simulink model "FusionMODEL_version4"  (R2018a)
settings: Solver=FixedStepAuto  StartTime=0.0  StopTime=SimulationTime  FixedStep=SamplingTime  RelTol=1e-3
values from neighbouring files (symbols this model uses):
  ValidateGRID = true    [SensorFusion_Script0_main.m]
  ValidateLAYOUT = true    [SensorFusion_Script0_main.m]
  VisualizeCLUSTERING = true    [SensorFusion_Script0_main.m]
undefined symbols (not defined in the file or in its folder): ACTIVATE_CAM, ACTIVATE_RAD, CAM1_detTimeStamp, CAM1_MeasNoise, CAM1_objClassID, CAM1_PX, CAM1_PY, CAM1_VX, CAM1_VY, CAM2_detTimeStamp, CAM2_MeasNoise, CAM2_objClassID, CAM2_PX, CAM2_PY, CAM2_VX, CAM2_VY, CAM3_detTimeStamp, CAM3_MeasNoise, CAM3_objClassID, CAM3_PX, CAM3_PY, CAM3_VX, CAM3_VY, CAM4_detTimeStamp, CAM4_MeasNoise, CAM4_objClassID, CAM4_PX, CAM4_PY, CAM4_VX, CAM4_VY, CAM5_detTimeStamp, CAM5_MeasNoise, CAM5_objClassID, CAM5_PX, CAM5_PY, CAM5_VX, CAM5_VY, CAM6_detTimeStamp, CAM6_MeasNoise, CAM6_objClassID, CAM6_PX, CAM6_PY, CAM6_VX, CAM6_VY, CAM7_detTimeStamp, CAM7_MeasNoise, CAM7_objClassID, CAM7_PX, CAM7_PY, CAM7_VX, CAM7_VY, CAM8_detTimeStamp, CAM8_MeasNoise, CAM8_objClassID, CAM8_PX, CAM8_PY, CAM8_VX, CAM8_VY, CAM_nMeas, CAM_TYPE ... (+171)
libraries: simulink_extras x4
(part 1 of 9)
settings Model: SimulationMode=accelerator  Creator=Udit Bhaskar  LastModifiedBy=Udit Bhaskar
settings OptimizationCC: EfficientMapNaN2IntZero=off
settings HardwareCC: TargetBitPerPointer=64  TargetBitPerSizeT=64  TargetBitPerPtrDiffT=64  TargetLongLongMode=on  TargetIntDivRoundTo=Zero  TargetEndianess=LittleEndian  TargetWordSize=64  TargetHWDeviceType=MATLAB Host  ProdEqTarget=off
settings CodeAppCC: MaxIdLength=128
settings GRTTargetCC: TargetLangStandard=C89/C90 (ANSI)  CombineOutputUpdateFcns=off  GRTInterface=on

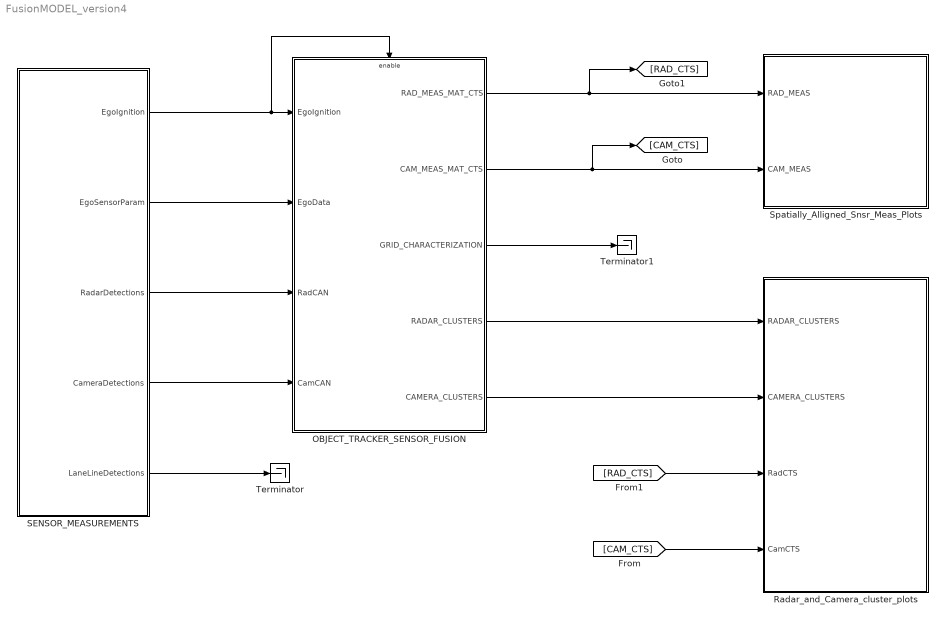
== system FusionMODEL_version4 ==
  OBJECT_TRACKER_SENSOR_FUSION : Subsystem
  Radar_and_Camera_cluster_plots : Subsystem
  SENSOR_MEASUREMENTS : Subsystem
  Spatially_Alligned_Snsr_Meas_Plots : Subsystem
  Terminator : Terminator
  Terminator1 : Terminator
  wires:
  SENSOR_MEASUREMENTS/5(LaneLineDetections) -> Terminator/1
  SENSOR_MEASUREMENTS/3(RadarDetections) -> OBJECT_TRACKER_SENSOR_FUSION/3(RadCAN)
  SENSOR_MEASUREMENTS/4(CameraDetections) -> OBJECT_TRACKER_SENSOR_FUSION/4(CamCAN)
  OBJECT_TRACKER_SENSOR_FUSION/1(RAD_MEAS_MAT_CTS) -> [RAD_CTS], Spatially_Alligned_Snsr_Meas_Plots/1(RAD_MEAS)
  OBJECT_TRACKER_SENSOR_FUSION/2(CAM_MEAS_MAT_CTS) -> [CAM_CTS], Spatially_Alligned_Snsr_Meas_Plots/2(CAM_MEAS)
  OBJECT_TRACKER_SENSOR_FUSION/3(GRID_CHARACTERIZATION) -> Terminator1/1
  SENSOR_MEASUREMENTS/1(EgoIgnition) -> OBJECT_TRACKER_SENSOR_FUSION/Enable, OBJECT_TRACKER_SENSOR_FUSION/1(EgoIgnition)
  OBJECT_TRACKER_SENSOR_FUSION/4(RADAR_CLUSTERS) -> Radar_and_Camera_cluster_plots/1(RADAR_CLUSTERS)
  OBJECT_TRACKER_SENSOR_FUSION/5(CAMERA_CLUSTERS) -> Radar_and_Camera_cluster_plots/2(CAMERA_CLUSTERS)
  [CAM_CTS] -> Radar_and_Camera_cluster_plots/4(CamCTS)
  [RAD_CTS] -> Radar_and_Camera_cluster_plots/3(RadCTS)
  SENSOR_MEASUREMENTS/2(EgoSensorParam) -> OBJECT_TRACKER_SENSOR_FUSION/2(EgoData)

== system FusionMODEL_version4/OBJECT_TRACKER_SENSOR_FUSION ==
  EgoIgnition : Inport
  EgoData : Inport  Port=2
  RadCAN : Inport  Port=3
  CamCAN : Inport  Port=4
  Enable : EnablePort
  NEAREST_NEIGHBOUR_FOR_CAMERA_MEASUREMENT_GROUPING : Subsystem
  SENSOR_LAYOUT_AND_CHRACTERIZATION : Subsystem
  SIMPLIFIED_DBSCAN_FOR_RADAR_MEASUREMENT_GROUPING : Subsystem
  SPATIAL_ALLIGNMENT : Subsystem
  Terminator : Terminator
  Unit Delay : UnitDelay  InitialCondition=false  SampleTime=-1
  RAD_MEAS_MAT_CTS : Outport
  CAM_MEAS_MAT_CTS : Outport  Port=2
  GRID_CHARACTERIZATION : Outport  Port=3
  RADAR_CLUSTERS : Outport  Port=4
  CAMERA_CLUSTERS : Outport  Port=5
  wires:
  SPATIAL_ALLIGNMENT/1(RadarMeasTransformed) -> RAD_MEAS_MAT_CTS/1, SIMPLIFIED_DBSCAN_FOR_RADAR_MEASUREMENT_GROUPING/1(RADAR_MEAS)
  RadCAN/1 -> SPATIAL_ALLIGNMENT/3(RadarCAN)
  SPATIAL_ALLIGNMENT/2(CameraMeasTransformed) -> NEAREST_NEIGHBOUR_FOR_CAMERA_MEASUREMENT_GROUPING/1(CAMERA_MEAS), CAM_MEAS_MAT_CTS/1
  CamCAN/1 -> SPATIAL_ALLIGNMENT/4(CameraCAN)
  SENSOR_LAYOUT_AND_CHRACTERIZATION/1(RAD_SNSR_PARAM) -> SPATIAL_ALLIGNMENT/1(RadarCallibrationParam)
  SENSOR_LAYOUT_AND_CHRACTERIZATION/2(CAM_SNSR_PARAM) -> SPATIAL_ALLIGNMENT/2(CameraCallibrationParam)
  SENSOR_LAYOUT_AND_CHRACTERIZATION/3(GRID_CHARACTERIZATION) -> GRID_CHARACTERIZATION/1
  EgoIgnition/1 -> Unit Delay/1
  Unit Delay/1 -> SENSOR_LAYOUT_AND_CHRACTERIZATION/Trigger
  SIMPLIFIED_DBSCAN_FOR_RADAR_MEASUREMENT_GROUPING/1(RADAR_CLUSTERS) -> RADAR_CLUSTERS/1
  NEAREST_NEIGHBOUR_FOR_CAMERA_MEASUREMENT_GROUPING/1(CAMERA_CLUSTERS) -> CAMERA_CLUSTERS/1
  EgoData/1 -> Terminator/1

== system FusionMODEL_version4/Radar_and_Camera_cluster_plots ==
  RADAR_CLUSTERS : Inport
  CAMERA_CLUSTERS : Inport  Port=2
  RadCTS : Inport  Port=3
  CamCTS : Inport  Port=4
  CAMERA : Subsystem
  Constant1 : Constant  Value=VisualizeCLUSTERING
  RADAR : Subsystem
  VISUALIZE_CLUSTERING : Subsystem
  wires:
  RADAR_CLUSTERS/1 -> VISUALIZE_CLUSTERING/1(In1), RADAR/1(In1)
  CAMERA_CLUSTERS/1 -> VISUALIZE_CLUSTERING/4(In4), CAMERA/1(In1)
  RadCTS/1 -> VISUALIZE_CLUSTERING/2(In2)
  CamCTS/1 -> VISUALIZE_CLUSTERING/3(In3)
  Constant1/1 -> VISUALIZE_CLUSTERING/Enable

== system FusionMODEL_version4/SENSOR_MEASUREMENTS ==
  RADAR_CAMERA_EGO_SENSOR_INTERFACE : Subsystem
  Subsystem : Subsystem
  Subsystem1 : Subsystem
  EgoIgnition : Outport
  EgoSensorParam : Outport  Port=2
  RadarDetections : Outport  Port=3
  CameraDetections : Outport  Port=4
  LaneLineDetections : Outport  Port=5
  wires:
  RADAR_CAMERA_EGO_SENSOR_INTERFACE/11(C5) -> Subsystem/11(C5)
  RADAR_CAMERA_EGO_SENSOR_INTERFACE/4(R4) -> Subsystem/4(R4)
  RADAR_CAMERA_EGO_SENSOR_INTERFACE/2(R2) -> Subsystem/2(R2)
  RADAR_CAMERA_EGO_SENSOR_INTERFACE/5(R5) -> Subsystem/5(R5)
  RADAR_CAMERA_EGO_SENSOR_INTERFACE/6(R6) -> Subsystem/6(R6)
  RADAR_CAMERA_EGO_SENSOR_INTERFACE/1(R1) -> Subsystem/1(R1)
  Subsystem/1(RadarMeasurementCAN) -> RadarDetections/1
  RADAR_CAMERA_EGO_SENSOR_INTERFACE/9(C3) -> Subsystem/9(C3)
  RADAR_CAMERA_EGO_SENSOR_INTERFACE/8(C2) -> Subsystem/8(C2)
  RADAR_CAMERA_EGO_SENSOR_INTERFACE/3(R3) -> Subsystem/3(R3)
  RADAR_CAMERA_EGO_SENSOR_INTERFACE/13(C7) -> Subsystem/13(C7)
  RADAR_CAMERA_EGO_SENSOR_INTERFACE/7(C1) -> Subsystem/7(C1)
  RADAR_CAMERA_EGO_SENSOR_INTERFACE/10(C4) -> Subsystem/10(C4)
  RADAR_CAMERA_EGO_SENSOR_INTERFACE/12(C6) -> Subsystem/12(C6)
  Subsystem/2(CameraMeasurementCAN) -> CameraDetections/1
  RADAR_CAMERA_EGO_SENSOR_INTERFACE/14(C8) -> Subsystem/14(C8)
  RADAR_CAMERA_EGO_SENSOR_INTERFACE/15(CAM_LINE1) -> Subsystem1/1(CAM_LINE1)
  RADAR_CAMERA_EGO_SENSOR_INTERFACE/16(CAM_LINE2) -> Subsystem1/2(CAM_LINE2)
  RADAR_CAMERA_EGO_SENSOR_INTERFACE/17(CAM_LINE3) -> Subsystem1/3(CAM_LINE3)
  RADAR_CAMERA_EGO_SENSOR_INTERFACE/18(CAM_LINE4) -> Subsystem1/4(CAM_LINE4)
  RADAR_CAMERA_EGO_SENSOR_INTERFACE/19(CAM_LINE5) -> Subsystem1/5(CAM_LINE5)
  RADAR_CAMERA_EGO_SENSOR_INTERFACE/20(CAM_LINE6) -> Subsystem1/6(CAM_LINE6)
  RADAR_CAMERA_EGO_SENSOR_INTERFACE/21(CAM_LINE7) -> Subsystem1/7(CAM_LINE7)
  RADAR_CAMERA_EGO_SENSOR_INTERFACE/22(CAM_LINE8) -> Subsystem1/8(CAM_LINE8)
  Subsystem1/1(LineMeasurementsCAN) -> LaneLineDetections/1
  RADAR_CAMERA_EGO_SENSOR_INTERFACE/23(EGO) -> EgoSensorParam/1
  RADAR_CAMERA_EGO_SENSOR_INTERFACE/24(EgoIgnition) -> EgoIgnition/1

== system FusionMODEL_version4/Spatially_Alligned_Snsr_Meas_Plots ==
  RAD_MEAS : Inport
  CAM_MEAS : Inport  Port=2
  Bus Selector : BusSelector  OutputSignals=MeasArray,ValidCumulativeMeasCount
  Bus Selector1 : BusSelector  OutputSignals=MeasArray,ValidCumulativeMeasCount
  CameraMeasCTS : Scope
  RadarMeasCTS : Scope
  Selector : Selector  NumberOfDimensions=2  InputPortWidth=3  IndexOptions=Select all,Index vector (port)  Indices=[1 3],1  OutputSizes=1,1
  Selector1 : Selector  NumberOfDimensions=2  InputPortWidth=3  IndexOptions=Index vector (dialog),Index vector (dialog)  Indices=1,1:30  OutputSizes=1,1
  Selector2 : Selector  NumberOfDimensions=2  InputPortWidth=3  IndexOptions=Select all,Index vector (port)  Indices=[1 3],1  OutputSizes=1,1
  Selector3 : Selector  NumberOfDimensions=2  InputPortWidth=3  IndexOptions=Index vector (dialog),Index vector (dialog)  Indices=1,1:30  OutputSizes=1,1
  Width : Width
  Width1 : Width
  nCameraMeasurements : Scope
  nRadarMeasurements : Scope
  wires:
  Bus Selector/1 -> Selector1/1  "<MeasArray>"
  Bus Selector/2 -> Selector/1, Width/1  "<ValidCumulativeMeasCount>"
  Width/1 -> Selector/2
  Selector1/1 -> RadarMeasCTS/1
  RAD_MEAS/1 -> Bus Selector/1
  Selector/1 -> nRadarMeasurements/1
  Bus Selector1/1 -> Selector3/1  "<MeasArray>"
  CAM_MEAS/1 -> Bus Selector1/1
  Width1/1 -> Selector2/2
  Selector2/1 -> nCameraMeasurements/1
  Selector3/1 -> CameraMeasCTS/1
  Bus Selector1/2 -> Selector2/1, Width1/1  "<ValidCumulativeMeasCount>"

== system FusionMODEL_version4/OBJECT_TRACKER_SENSOR_FUSION/NEAREST_NEIGHBOUR_FOR_CAMERA_MEASUREMENT_GROUPING ==
  CAMERA_MEAS : Inport
  GET_NUM_OF_MEAS : Subsystem
  NN_MEASUREMENT_GROUPING_WITHIN_EPS : Subsystem  TreatAsAtomicUnit=on
  CAMERA_CLUSTERS : Outport
  wires:
  GET_NUM_OF_MEAS/1(nMeas) -> NN_MEASUREMENT_GROUPING_WITHIN_EPS/1(nMeas)
  CAMERA_MEAS/1 -> GET_NUM_OF_MEAS/1(CAM_MEAS_CTS), NN_MEASUREMENT_GROUPING_WITHIN_EPS/2(Meas)
  NN_MEASUREMENT_GROUPING_WITHIN_EPS/1(CAMERA_CLUSTERS) -> CAMERA_CLUSTERS/1

== system FusionMODEL_version4/OBJECT_TRACKER_SENSOR_FUSION/SENSOR_LAYOUT_AND_CHRACTERIZATION ==
  Trigger : TriggerPort  VariantControl=Variant  PortDimensions=1
  Constant : Constant  Value=ValidateGRID
  Constant1 : Constant  Value=ValidateLAYOUT
  Ground1 : Ground
  Ground2 : Ground
  PRE_COMPUTE_SENSOR_FOV_GRID : Subsystem
  SET_SENSOR_CALLIBRATION_PARAMETER : Subsystem
  ValidateGrid : Subsystem
  ValidateSensorLayout : Subsystem
  RAD_SNSR_PARAM : Outport
  CAM_SNSR_PARAM : Outport  Port=2
  GRID_CHARACTERIZATION : Outport  Port=3
  wires:
  SET_SENSOR_CALLIBRATION_PARAMETER/2(CameraCalibParamUpd) -> [CAM_SNSR_PARAM], CAM_SNSR_PARAM/1, PRE_COMPUTE_SENSOR_FOV_GRID/2(CAMSnsrParam)
  Ground2/1 -> SET_SENSOR_CALLIBRATION_PARAMETER/2(RADSnsrParam)
  Ground1/1 -> SET_SENSOR_CALLIBRATION_PARAMETER/1(CamCalibParam)
  SET_SENSOR_CALLIBRATION_PARAMETER/1(RadarCalibParamUpd) -> RAD_SNSR_PARAM/1, [RAD_SNSR_PARAM], PRE_COMPUTE_SENSOR_FOV_GRID/1(RADSnsrParam)
  PRE_COMPUTE_SENSOR_FOV_GRID/1(GRID_CHARACTERIZATION) -> [GRID], GRID_CHARACTERIZATION/1
  Constant/1 -> ValidateGrid/Enable
  [RAD_SNSR_PARAM] -> ValidateSensorLayout/1(RAD_SNSR_PARAM)
  [CAM_SNSR_PARAM] -> ValidateSensorLayout/2(CAM_SNSR_PARAM)
  [GRID] -> ValidateGrid/1(In1)
  Constant1/1 -> ValidateSensorLayout/Enable

== system FusionMODEL_version4/OBJECT_TRACKER_SENSOR_FUSION/SIMPLIFIED_DBSCAN_FOR_RADAR_MEASUREMENT_GROUPING ==
  RADAR_MEAS : Inport
  DBSCAN_MEASUREMENT_GROUPING : Subsystem  TreatAsAtomicUnit=on
  GET_NUM_OF_MEAS : Subsystem
  RADAR_CLUSTERS : Outport
  wires:
  GET_NUM_OF_MEAS/1(nMeas) -> DBSCAN_MEASUREMENT_GROUPING/1(nMeas)
  RADAR_MEAS/1 -> GET_NUM_OF_MEAS/1(RAD_MEAS_CTS), DBSCAN_MEASUREMENT_GROUPING/2(Meas)
  DBSCAN_MEASUREMENT_GROUPING/1(RADAR_CLUSTERS) -> RADAR_CLUSTERS/1

== system FusionMODEL_version4/OBJECT_TRACKER_SENSOR_FUSION/SPATIAL_ALLIGNMENT ==
  RadarCallibrationParam : Inport
  CameraCallibrationParam : Inport  Port=2
  RadarCAN : Inport  Port=3
  CameraCAN : Inport  Port=4
  CAMERA_MEASUREMENTS_SPATIAL_ALLIGNMENT : Subsystem
  GET_CAM_MEAS : Subsystem
  GET_RAD_MEAS : Subsystem
  RADAR_MEASUREMENTS_SPATIAL_ALLIGNMENT : Subsystem
  RadarMeasTransformed : Outport
  CameraMeasTransformed : Outport  Port=2
  wires:
  RadarCAN/1 -> GET_RAD_MEAS/2(RadarMeas)
  CameraCAN/1 -> GET_CAM_MEAS/2(CameraMeas)
  GET_CAM_MEAS/2(<C1>) -> CAMERA_MEASUREMENTS_SPATIAL_ALLIGNMENT/2(C1)
  GET_CAM_MEAS/3(<C2>) -> CAMERA_MEASUREMENTS_SPATIAL_ALLIGNMENT/3(C2)
  GET_CAM_MEAS/4(<C3>) -> CAMERA_MEASUREMENTS_SPATIAL_ALLIGNMENT/4(C3)
  GET_CAM_MEAS/5(<C4>) -> CAMERA_MEASUREMENTS_SPATIAL_ALLIGNMENT/5(C4)
  GET_CAM_MEAS/6(<C5>) -> CAMERA_MEASUREMENTS_SPATIAL_ALLIGNMENT/6(C5)
  GET_CAM_MEAS/7(<C6>) -> CAMERA_MEASUREMENTS_SPATIAL_ALLIGNMENT/7(C6)
  GET_CAM_MEAS/8(<C7>) -> CAMERA_MEASUREMENTS_SPATIAL_ALLIGNMENT/8(C7)
  GET_CAM_MEAS/9(<C8>) -> CAMERA_MEASUREMENTS_SPATIAL_ALLIGNMENT/9(C8)
  GET_RAD_MEAS/2(<R1>) -> RADAR_MEASUREMENTS_SPATIAL_ALLIGNMENT/2(R1)
  GET_RAD_MEAS/3(<R2>) -> RADAR_MEASUREMENTS_SPATIAL_ALLIGNMENT/3(R2)
  GET_RAD_MEAS/4(<R3>) -> RADAR_MEASUREMENTS_SPATIAL_ALLIGNMENT/4(R3)
  GET_RAD_MEAS/5(<R4>) -> RADAR_MEASUREMENTS_SPATIAL_ALLIGNMENT/5(R4)
  GET_RAD_MEAS/6(<R5>) -> RADAR_MEASUREMENTS_SPATIAL_ALLIGNMENT/6(R5)
  GET_RAD_MEAS/7(<R6>) -> RADAR_MEASUREMENTS_SPATIAL_ALLIGNMENT/7(R6)
  GET_RAD_MEAS/1(SnsrParam) -> RADAR_MEASUREMENTS_SPATIAL_ALLIGNMENT/1(RadarCalibParam)
  RadarCallibrationParam/1 -> GET_RAD_MEAS/1(RadarParam)
  GET_CAM_MEAS/1(SnsrParam) -> CAMERA_MEASUREMENTS_SPATIAL_ALLIGNMENT/1(CameraCalibParam)
  CameraCallibrationParam/1 -> GET_CAM_MEAS/1(CameraParam)
  CAMERA_MEASUREMENTS_SPATIAL_ALLIGNMENT/1(CameraMeasTransformed) -> CameraMeasTransformed/1
  RADAR_MEASUREMENTS_SPATIAL_ALLIGNMENT/1(RadarMeasTransformed) -> RadarMeasTransformed/1

== system FusionMODEL_version4/Radar_and_Camera_cluster_plots/CAMERA ==
  In1 : Inport
  Bus Selector : BusSelector  OutputSignals=ClusterSizes,nClusters,ClusterCenter
  Scope{,1..3} (4 alike) : Scope
  Selector : Selector  NumberOfDimensions=2  InputPortWidth=3  IndexOptions=Index vector (dialog),Index vector (dialog)  Indices=1,1:10  OutputSizes=1,1
  Selector1 : Selector  NumberOfDimensions=2  InputPortWidth=3  IndexOptions=Index vector (dialog),Index vector (dialog)  Indices=2,1:10  OutputSizes=1,1
  Selector2 : Selector  NumberOfDimensions=2  InputPortWidth=3  IndexOptions=Select all,Index vector (dialog)  Indices=[1 3],1:10  OutputSizes=1,1
  wires:
  Bus Selector/3 -> Selector/1, Selector1/1  "<ClusterCenter>"
  In1/1 -> Bus Selector/1
  Bus Selector/2 -> Scope/1  "<nClusters>"
  Bus Selector/1 -> Selector2/1  "<ClusterSizes>"
  Selector/1 -> Scope1/1
  Selector1/1 -> Scope3/1
  Selector2/1 -> Scope2/1

== system FusionMODEL_version4/Radar_and_Camera_cluster_plots/RADAR ==
  In1 : Inport
  Bus Selector1 : BusSelector  OutputSignals=ClusterSizes,nClusters,ClusterCenter
  Scope{1..4} (4 alike) : Scope
  Selector : Selector  NumberOfDimensions=2  InputPortWidth=3  IndexOptions=Select all,Index vector (dialog)  Indices=[1 3],1:10  OutputSizes=1,1
  Selector2 : Selector  NumberOfDimensions=2  InputPortWidth=3  IndexOptions=Index vector (dialog),Index vector (dialog)  Indices=1,1:10  OutputSizes=1,1
  Selector3 : Selector  NumberOfDimensions=2  InputPortWidth=3  IndexOptions=Index vector (dialog),Index vector (dialog)  Indices=2,1:10  OutputSizes=1,1
  wires:
  Bus Selector1/2 -> Scope1/1  "<nClusters>"
  Bus Selector1/3 -> Selector2/1, Selector3/1  "<ClusterCenter>"
  Bus Selector1/1 -> Selector/1  "<ClusterSizes>"
  Selector3/1 -> Scope4/1
  Selector2/1 -> Scope2/1
  In1/1 -> Bus Selector1/1
  Selector/1 -> Scope3/1

== system FusionMODEL_version4/Radar_and_Camera_cluster_plots/VISUALIZE_CLUSTERING ==
  In1 : Inport
  In2 : Inport  Port=2
  In3 : Inport  Port=3
  In4 : Inport  Port=4
  Enable : EnablePort
  MATLAB Function : MATLAB Function  TreatAsAtomicUnit=on
  wires:
  In2/1 -> MATLAB Function/2(RadMeas)
  In1/1 -> MATLAB Function/1(RadCluster)
  In4/1 -> MATLAB Function/4(CamCluster)
  In3/1 -> MATLAB Function/3(CamMeas)

== system FusionMODEL_version4/SENSOR_MEASUREMENTS/RADAR_CAMERA_EGO_SENSOR_INTERFACE ==
  CameraSensors : Subsystem
  Clock : Subsystem
  EgoSensors : Subsystem
  Ground{,1..3} (4 alike) : Ground
  RadarSensors : Subsystem
  RoadSensors : Subsystem
  R1 : Outport
  R2 : Outport  Port=2
  R3 : Outport  Port=3
  R4 : Outport  Port=4
  R5 : Outport  Port=5
  R6 : Outport  Port=6
  C1 : Outport  Port=7
  C2 : Outport  Port=8
  C3 : Outport  Port=9
  C4 : Outport  Port=10
  C5 : Outport  Port=11
  C6 : Outport  Port=12
  C7 : Outport  Port=13
  C8 : Outport  Port=14
  CAM_LINE1 : Outport  Port=15
  CAM_LINE2 : Outport  Port=16
  CAM_LINE3 : Outport  Port=17
  CAM_LINE4 : Outport  Port=18
  CAM_LINE5 : Outport  Port=19
  CAM_LINE6 : Outport  Port=20
  CAM_LINE7 : Outport  Port=21
  CAM_LINE8 : Outport  Port=22
  EGO : Outport  Port=23
  EgoIgnition : Outport  Port=24
  wires:
  RadarSensors/6(R6) -> R6/1
  RadarSensors/4(R4) -> R4/1
  Clock/2(nObjRadar) -> RadarSensors/2(nObjRadar)
  Clock/3(nObjCamera) -> CameraSensors/2(nObjCamera)
  CameraSensors/3(C3) -> C3/1
  RadarSensors/5(R5) -> R5/1
  CameraSensors/5(C5) -> C5/1
  CameraSensors/4(C4) -> C4/1
  CameraSensors/8(C8) -> C8/1
  CameraSensors/7(C7) -> C7/1
  CameraSensors/6(C6) -> C6/1
  CameraSensors/2(C2) -> C2/1
  RadarSensors/2(R2) -> R2/1
  RadarSensors/3(R3) -> R3/1
  CameraSensors/1(C1) -> C1/1
  RadarSensors/1(R1) -> R1/1
  Clock/1(time) -> CameraSensors/1(time), RoadSensors/1(time), EgoSensors/1(timeIdx), RadarSensors/1(time)
  Clock/4(nLinesCamera) -> RoadSensors/2(nLinesCamera)
  RoadSensors/1(C1) -> CAM_LINE1/1
  RoadSensors/2(C2) -> CAM_LINE2/1
  RoadSensors/3(C3) -> CAM_LINE3/1
  RoadSensors/4(C4) -> CAM_LINE4/1
  RoadSensors/5(C5) -> CAM_LINE5/1
  RoadSensors/6(C6) -> CAM_LINE6/1
  RoadSensors/7(C7) -> CAM_LINE7/1
  RoadSensors/8(C8) -> CAM_LINE8/1
  EgoSensors/1(EgoSensorData) -> EGO/1
  Ground1/1 -> RadarSensors/3(RADSensorBUS)
  Ground2/1 -> CameraSensors/3(CAMSensorBUS)
  Ground/1 -> EgoSensors/2(In1)
  Ground3/1 -> RoadSensors/3(CameraLineCoeff1)
  EgoSensors/2(EgoIgnitionStatus) -> EgoIgnition/1

== system FusionMODEL_version4/SENSOR_MEASUREMENTS/Subsystem ==
  R1 : Inport
  R2 : Inport  Port=2
  R3 : Inport  Port=3
  R4 : Inport  Port=4
  R5 : Inport  Port=5
  R6 : Inport  Port=6
  C1 : Inport  Port=7
  C2 : Inport  Port=8
  C3 : Inport  Port=9
  C4 : Inport  Port=10
  C5 : Inport  Port=11
  C6 : Inport  Port=12
  C7 : Inport  Port=13
  C8 : Inport  Port=14
  Bus Creator : BusCreator  Inputs=6  OutDataTypeStr=Bus: RAD_MEAS_INTERFACE  NonVirtualBus=on
  Bus Creator1 : BusCreator  Inputs=8  OutDataTypeStr=Bus: CAM_MEAS_INTERFACE  NonVirtualBus=on
  RadarMeasurementCAN : Outport
  CameraMeasurementCAN : Outport  Port=2
  wires:
  R1/1 -> Bus Creator/1  "R1"
  R6/1 -> Bus Creator/6  "R6"
  R5/1 -> Bus Creator/5  "R5"
  R4/1 -> Bus Creator/4  "R4"
  R3/1 -> Bus Creator/3  "R3"
  R2/1 -> Bus Creator/2  "R2"
  Bus Creator/1 -> RadarMeasurementCAN/1
  C1/1 -> Bus Creator1/1  "C1"
  C2/1 -> Bus Creator1/2  "C2"
  C3/1 -> Bus Creator1/3  "C3"
  C4/1 -> Bus Creator1/4  "C4"
  C5/1 -> Bus Creator1/5  "C5"
  C6/1 -> Bus Creator1/6  "C6"
  C7/1 -> Bus Creator1/7  "C7"
  C8/1 -> Bus Creator1/8  "C8"
  Bus Creator1/1 -> CameraMeasurementCAN/1

== system FusionMODEL_version4/SENSOR_MEASUREMENTS/Subsystem1 ==
  CAM_LINE1 : Inport
  CAM_LINE2 : Inport  Port=2
  CAM_LINE3 : Inport  Port=3
  CAM_LINE4 : Inport  Port=4
  CAM_LINE5 : Inport  Port=5
  CAM_LINE6 : Inport  Port=6
  CAM_LINE7 : Inport  Port=7
  CAM_LINE8 : Inport  Port=8
  Bus Creator : BusCreator  Inputs=8  OutDataTypeStr=Bus: LINE_MEAS_INTERFACE  NonVirtualBus=on
  LineMeasurementsCAN : Outport
  wires:
  CAM_LINE1/1 -> Bus Creator/1  "C1_LINE"
  CAM_LINE2/1 -> Bus Creator/2  "C2_LINE"
  CAM_LINE3/1 -> Bus Creator/3  "C3_LINE"
  CAM_LINE4/1 -> Bus Creator/4  "C4_LINE"
  CAM_LINE5/1 -> Bus Creator/5  "C5_LINE"
  CAM_LINE6/1 -> Bus Creator/6  "C6_LINE"
  CAM_LINE7/1 -> Bus Creator/7  "C7_LINE"
  CAM_LINE8/1 -> Bus Creator/8  "C8_LINE"
  Bus Creator/1 -> LineMeasurementsCAN/1

== system FusionMODEL_version4/OBJECT_TRACKER_SENSOR_FUSION/NEAREST_NEIGHBOUR_FOR_CAMERA_MEASUREMENT_GROUPING/GET_NUM_OF_MEAS ==
  CAM_MEAS_CTS : Inport
  Bus Selector : BusSelector  OutputSignals=ValidCumulativeMeasCount
  Selector : Selector  NumberOfDimensions=2  InputPortWidth=3  IndexOptions=Select all,Index vector (port)  Indices=[1 3],1  OutputSizes=1,1
  Width : Width
  nMeas : Outport
  wires:
  CAM_MEAS_CTS/1 -> Bus Selector/1
  Bus Selector/1 -> Width/1, Selector/1  "<ValidCumulativeMeasCount>"
  Selector/1 -> nMeas/1
  Width/1 -> Selector/2

== system FusionMODEL_version4/OBJECT_TRACKER_SENSOR_FUSION/NEAREST_NEIGHBOUR_FOR_CAMERA_MEASUREMENT_GROUPING/NN_MEASUREMENT_GROUPING_WITHIN_EPS ==
  nMeas : Inport
  Meas : Inport  Port=2
  COMPUTE_MEAN_IF_CLUSTER_FORMED : Subsystem
  For Iterator : ForIterator  ResetStates=reset  IterationSource=external
  For Iterator Subsystem : Subsystem  TreatAsAtomicUnit=on
  Subsystem1 : Subsystem
  Subsystem2 : Subsystem
  Subsystem3 : Subsystem
  CAMERA_CLUSTERS : Outport
  wires:
  nMeas/1 -> For Iterator/1
  For Iterator/1 -> For Iterator Subsystem/1(idx_i)
  Meas/1 -> [meas], For Iterator Subsystem/2(measArray)
  For Iterator Subsystem/2(CLSTR_DATA_out) -> COMPUTE_MEAN_IF_CLUSTER_FORMED/2(CLSTR_DATA), Subsystem3/5(CLSTR_DATA)
  Subsystem1/2(Upd) -> COMPUTE_MEAN_IF_CLUSTER_FORMED/Enable
  Subsystem1/1(NoUpd) -> Subsystem2/Enable
  COMPUTE_MEAN_IF_CLUSTER_FORMED/1(CLSTR_CNTR_UPD) -> Subsystem3/3(MeanUpd)
  Subsystem2/1(Mean) -> Subsystem3/1(MeanNoUpd)
  Subsystem2/2(Cov) -> Subsystem3/2(CovNoUpd)
  COMPUTE_MEAN_IF_CLUSTER_FORMED/2(CLSTR_COV_UPD) -> Subsystem3/4(CovUpd)
  Subsystem3/1(CLSTR_DATA_UPD) -> CAMERA_CLUSTERS/1, For Iterator Subsystem/3(CLSTR_DATA)
  [A] -> Subsystem3/6(Flag)
  For Iterator Subsystem/1(nPts) -> [A], Subsystem1/1(CLSTR_DATA)
  [meas] -> COMPUTE_MEAN_IF_CLUSTER_FORMED/1(meas)

== system FusionMODEL_version4/OBJECT_TRACKER_SENSOR_FUSION/SENSOR_LAYOUT_AND_CHRACTERIZATION/PRE_COMPUTE_SENSOR_FOV_GRID ==
  RADSnsrParam : Inport
  CAMSnsrParam : Inport  Port=2
  COMPUTE_CAMERA_SNSR_GRID : Subsystem
  COMPUTE_GRID_DIMENSION : Subsystem
  COMPUTE_RADAR_SNSR_GRID : Subsystem
  CREATE_GRID : Subsystem  TreatAsAtomicUnit=on
  SET_DATA : Subsystem
  GRID_CHARACTERIZATION : Outport
  wires:
  RADSnsrParam/1 -> COMPUTE_RADAR_SNSR_GRID/1(SnsrParam)
  COMPUTE_GRID_DIMENSION/2(Cy) -> CREATE_GRID/2(Cy)
  COMPUTE_GRID_DIMENSION/3(GridParam) -> [GridParam], CREATE_GRID/3(GridParam)
  COMPUTE_GRID_DIMENSION/1(Cx) -> CREATE_GRID/1(Cx)
  CREATE_GRID/1(CellIDVectorUpd) -> COMPUTE_CAMERA_SNSR_GRID/1(GridIDVector), COMPUTE_RADAR_SNSR_GRID/3(GridIDVector)
  [GridParam] -> COMPUTE_RADAR_SNSR_GRID/2(GridParam)
  [GridParam] -> COMPUTE_CAMERA_SNSR_GRID/2(GridParam)
  CAMSnsrParam/1 -> COMPUTE_CAMERA_SNSR_GRID/3(SnsrParam)
  [GridParam] -> SET_DATA/1(GRID_PARAM)  "GRID_PARAM"
  COMPUTE_RADAR_SNSR_GRID/1(RegionConfidence) -> SET_DATA/2(RAD_REGION_CONFIDENCE)  "RAD_REGION_CONFIDENCE"
  COMPUTE_RADAR_SNSR_GRID/2(FOVOverlap) -> SET_DATA/3(RAD_FOV_OVERLAP)  "RAD_FOV_OVERLAP"
  COMPUTE_CAMERA_SNSR_GRID/1(RegionConfidence) -> SET_DATA/4(CAM_REGION_CONFIDENCE)  "CAM_REGION_CONFIDENCE"
  COMPUTE_CAMERA_SNSR_GRID/2(FOVOverlap) -> SET_DATA/5(CAM_FOV_OVERLAP)  "CAM_FOV_OVERLAP"
  SET_DATA/1(GRID_CHARACTERIZATION) -> GRID_CHARACTERIZATION/1

== system FusionMODEL_version4/OBJECT_TRACKER_SENSOR_FUSION/SENSOR_LAYOUT_AND_CHRACTERIZATION/SET_SENSOR_CALLIBRATION_PARAMETER ==
  CamCalibParam : Inport  OutDataTypeStr=Bus: CAM_SENSOR_PARAM  PortDimensions=nCameraActive  BusOutputAsStruct=on
  RADSnsrParam : Inport  Port=2  OutDataTypeStr=Bus: RAD_SENSOR_PARAM  PortDimensions=1
  SET_CAMERA_SENSOR_PARAM : Subsystem  TreatAsAtomicUnit=on
  SET_RADAR_SENSOR_PARAM : Subsystem
  RadarCalibParamUpd : Outport
  CameraCalibParamUpd : Outport  Port=2
  wires:
  SET_CAMERA_SENSOR_PARAM/1(CAMSnsrParamUpd) -> CameraCalibParamUpd/1
  CamCalibParam/1 -> SET_CAMERA_SENSOR_PARAM/1(CAMSnsrParam)
  RADSnsrParam/1 -> SET_RADAR_SENSOR_PARAM/1(RADSnsrParam)
  SET_RADAR_SENSOR_PARAM/1(RADSnsrParamUpd) -> RadarCalibParamUpd/1

== system FusionMODEL_version4/OBJECT_TRACKER_SENSOR_FUSION/SENSOR_LAYOUT_AND_CHRACTERIZATION/ValidateGrid ==
  In1 : Inport
  Enable : EnablePort
  Bus Selector : BusSelector  OutputSignals=GRID_PARAM,RAD_GRID,CAM_GRID
  Bus Selector1 : BusSelector  OutputSignals=xGridParameters,yGridParameters
  Bus Selector2 : BusSelector  OutputSignals=nGridCellsLong,xRes,xFront,xRear
  Bus Selector3 : BusSelector  OutputSignals=nGridCellsLat,yRes,yRight,yLeft
  Bus Selector4 : BusSelector  OutputSignals=RAD_REGION_CONFIDENCE,RAD_FOV_OVERLAP
  Bus Selector5 : BusSelector  OutputSignals=CAM_REGION_CONFIDENCE,CAM_FOV_OVERLAP
  MATLAB Function : MATLAB Function  TreatAsAtomicUnit=on
  To Workspace : ToWorkspace  VariableName=HeatMapRAD_FOV  SaveFormat=Timeseries  SampleTime=-1
  To Workspace1 : ToWorkspace  VariableName=HeatMapCAM_FOV  SaveFormat=Timeseries  SampleTime=-1
  To Workspace2 : ToWorkspace  VariableName=HeatMapCAM_CONFI  SaveFormat=Timeseries  SampleTime=-1
  To Workspace3 : ToWorkspace  VariableName=HeatMapRAD_CONFI  SaveFormat=Timeseries  SampleTime=-1
  To Workspace4 : ToWorkspace  VariableName=HeatMap_RAD_CAM_FOV  SaveFormat=Timeseries  SampleTime=-1
  To Workspace5 : ToWorkspace  VariableName=HeatMap_RAD_CAM_CONFI  SaveFormat=Timeseries  SampleTime=-1
  wires:
  In1/1 -> Bus Selector/1
  Bus Selector/1 -> Bus Selector1/1  "<GRID_PARAM>"
  Bus Selector1/1 -> Bus Selector2/1  "<xGridParameters>"
  Bus Selector1/2 -> Bus Selector3/1  "<yGridParameters>"
  Bus Selector/2 -> Bus Selector4/1  "<RAD_GRID>"
  Bus Selector/3 -> Bus Selector5/1  "<CAM_GRID>"
  Bus Selector2/1 -> MATLAB Function/1(Cx)  "<nGridCellsLong>"
  Bus Selector2/2 -> MATLAB Function/2(dx)  "<xRes>"
  Bus Selector2/3 -> MATLAB Function/3(XUpperLimit)  "<xFront>"
  Bus Selector2/4 -> MATLAB Function/4(XLowerLimit)  "<xRear>"
  Bus Selector3/1 -> MATLAB Function/5(Cy)  "<nGridCellsLat>"
  Bus Selector3/2 -> MATLAB Function/6(dy)  "<yRes>"
  Bus Selector3/3 -> MATLAB Function/7(YUpperLimit)  "<yRight>"
  Bus Selector3/4 -> MATLAB Function/8(YLowerLimit)  "<yLeft>"
  Bus Selector4/1 -> MATLAB Function/9(RADAR_GRID_CONFI)  "<RAD_REGION_CONFIDENCE>"
  Bus Selector4/2 -> MATLAB Function/10(RADAR_GRID_FOV)  "<RAD_FOV_OVERLAP>"
  Bus Selector5/1 -> MATLAB Function/11(CAMERA_GRID_CONFI)  "<CAM_REGION_CONFIDENCE>"
  Bus Selector5/2 -> MATLAB Function/12(CAMERA_GRID_FOV)  "<CAM_FOV_OVERLAP>"
  MATLAB Function/1(HeatMapRAD_FOV) -> To Workspace/1
  MATLAB Function/3(HeatMapCAM_FOV) -> To Workspace1/1
  MATLAB Function/4(HeatMapCAM_CONFI) -> To Workspace2/1
  MATLAB Function/2(HeatMapRAD_CONFI) -> To Workspace3/1
  MATLAB Function/5(HeatMap_RAD_CAM_FOV) -> To Workspace4/1
  MATLAB Function/6(HeatMap_RAD_CAM_CONFI) -> To Workspace5/1

== system FusionMODEL_version4/OBJECT_TRACKER_SENSOR_FUSION/SENSOR_LAYOUT_AND_CHRACTERIZATION/ValidateSensorLayout ==
  RAD_SNSR_PARAM : Inport
  CAM_SNSR_PARAM : Inport  Port=2
  Enable : EnablePort
  MATLAB Function : MATLAB Function  TreatAsAtomicUnit=on
  wires:
  RAD_SNSR_PARAM/1 -> MATLAB Function/1(RadarParam)
  CAM_SNSR_PARAM/1 -> MATLAB Function/2(CameraParam)

== system FusionMODEL_version4/OBJECT_TRACKER_SENSOR_FUSION/SIMPLIFIED_DBSCAN_FOR_RADAR_MEASUREMENT_GROUPING/DBSCAN_MEASUREMENT_GROUPING ==
  nMeas : Inport
  Meas : Inport  Port=2
  CHECK_IF_CLUSTER_FORMED : Subsystem
  COMPUTE_MEAN_IF_CLUSTER_FORMED : Subsystem
  FORM_CLUSTER : Subsystem  TreatAsAtomicUnit=on
  For Iterator : ForIterator  ResetStates=reset  IterationSource=external
  IF_CLUSTER_NOT_FORMED : Subsystem
  MERGE_SIGNALS : Subsystem
  RADAR_CLUSTERS : Outport
  wires:
  nMeas/1 -> For Iterator/1
  For Iterator/1 -> FORM_CLUSTER/1(idx_i)
  Meas/1 -> [meas], FORM_CLUSTER/2(measArray)
  FORM_CLUSTER/2(isMeasVisited) -> COMPUTE_MEAN_IF_CLUSTER_FORMED/1(CLSTR_DATA), MERGE_SIGNALS/5(CLSTR_DATA)
  CHECK_IF_CLUSTER_FORMED/2(Upd) -> COMPUTE_MEAN_IF_CLUSTER_FORMED/Enable
  CHECK_IF_CLUSTER_FORMED/1(NoUpd) -> IF_CLUSTER_NOT_FORMED/Enable
  COMPUTE_MEAN_IF_CLUSTER_FORMED/1(CLSTR_CNTR_UPD) -> MERGE_SIGNALS/3(MeanUpd)
  IF_CLUSTER_NOT_FORMED/1(Mean) -> MERGE_SIGNALS/1(MeanNoUpd)
  IF_CLUSTER_NOT_FORMED/2(Cov) -> MERGE_SIGNALS/2(CovNoUpd)
  COMPUTE_MEAN_IF_CLUSTER_FORMED/2(CLSTR_COV_UPD) -> MERGE_SIGNALS/4(CovUpd)
  MERGE_SIGNALS/1(CLSTR_DATA_UPD) -> RADAR_CLUSTERS/1, FORM_CLUSTER/3(CLSTR_DATA)
  [meas] -> COMPUTE_MEAN_IF_CLUSTER_FORMED/2(meas)
  [A] -> MERGE_SIGNALS/6(Flag)
  FORM_CLUSTER/1(nPts) -> [A], CHECK_IF_CLUSTER_FORMED/1(nPts)

== system FusionMODEL_version4/OBJECT_TRACKER_SENSOR_FUSION/SIMPLIFIED_DBSCAN_FOR_RADAR_MEASUREMENT_GROUPING/GET_NUM_OF_MEAS ==
  RAD_MEAS_CTS : Inport
  Bus Selector : BusSelector  OutputSignals=ValidCumulativeMeasCount
  Selector : Selector  NumberOfDimensions=2  InputPortWidth=3  IndexOptions=Select all,Index vector (port)  Indices=[1 3],1  OutputSizes=1,1
  Width : Width
  nMeas : Outport
  wires:
  RAD_MEAS_CTS/1 -> Bus Selector/1
  Bus Selector/1 -> Width/1, Selector/1  "<ValidCumulativeMeasCount>"
  Selector/1 -> nMeas/1
  Width/1 -> Selector/2

== system FusionMODEL_version4/OBJECT_TRACKER_SENSOR_FUSION/SPATIAL_ALLIGNMENT/CAMERA_MEASUREMENTS_SPATIAL_ALLIGNMENT ==
  CameraCalibParam : Inport  BusOutputAsStruct=on
  C1 : Inport  Port=2
  C2 : Inport  Port=3
  C3 : Inport  Port=4
  C4 : Inport  Port=5
  C5 : Inport  Port=6
  C6 : Inport  Port=7
  C7 : Inport  Port=8
  C8 : Inport  Port=9
  For Iterator Subsystem : Subsystem  TreatAsAtomicUnit=on
  RadarMeasurementIndexes2 : Subsystem
  StartingIndexes1 : Subsystem
  CameraMeasTransformed : Outport
  wires:
  CameraCalibParam/1 -> For Iterator Subsystem/1(CameraCallibrationParam), StartingIndexes1/1(SnsrCallib)
  C6/1 -> For Iterator Subsystem/8(C6)
  C3/1 -> For Iterator Subsystem/5(C3)
  C4/1 -> For Iterator Subsystem/6(C4)
  C2/1 -> For Iterator Subsystem/4(C2)
  C1/1 -> For Iterator Subsystem/3(C1)
  StartingIndexes1/1(StartingIndexes) -> For Iterator Subsystem/2(RadarStartingIdx)
  C5/1 -> For Iterator Subsystem/7(C5)
  C7/1 -> For Iterator Subsystem/9(C7)
  C8/1 -> For Iterator Subsystem/10(C8)
  For Iterator Subsystem/2(CameraMeasTransformed) -> RadarMeasurementIndexes2/2(CTSmeasMAT)
  RadarMeasurementIndexes2/1(CTSmeasMATout) -> CameraMeasTransformed/1
  For Iterator Subsystem/4(CameraMeasRef) -> RadarMeasurementIndexes2/4(CTSRefMAT)
  For Iterator Subsystem/3(CameraMeasCOVTransformed) -> RadarMeasurementIndexes2/3(CTSCovMAT)
  For Iterator Subsystem/1(MaxNoValidMeas) -> RadarMeasurementIndexes2/1(validMeasCount)

== system FusionMODEL_version4/OBJECT_TRACKER_SENSOR_FUSION/SPATIAL_ALLIGNMENT/GET_CAM_MEAS ==
  CameraParam : Inport
  CameraMeas : Inport  Port=2
  Bus Selector1 : BusSelector  OutputSignals=C1,C2,C3,C4,C5,C6,C7,C8
  Bus Selector2 : BusSelector  OutputSignals=CameraExtrinsics
  SnsrParam : Outport
  <C1> : Outport  Port=2
  <C2> : Outport  Port=3
  <C3> : Outport  Port=4
  <C4> : Outport  Port=5
  <C5> : Outport  Port=6
  <C6> : Outport  Port=7
  <C7> : Outport  Port=8
  <C8> : Outport  Port=9
  wires:
  Bus Selector1/4 -> <C4>/1  "<C4>"
  Bus Selector1/6 -> <C6>/1  "<C6>"
  Bus Selector1/5 -> <C5>/1  "<C5>"
  CameraMeas/1 -> Bus Selector1/1
  Bus Selector1/1 -> <C1>/1  "<C1>"
  Bus Selector1/7 -> <C7>/1  "<C7>"
  Bus Selector1/8 -> <C8>/1  "<C8>"
  Bus Selector1/2 -> <C2>/1  "<C2>"
  Bus Selector1/3 -> <C3>/1  "<C3>"
  CameraParam/1 -> Bus Selector2/1
  Bus Selector2/1 -> SnsrParam/1  "<CameraExtrinsics>"

== system FusionMODEL_version4/OBJECT_TRACKER_SENSOR_FUSION/SPATIAL_ALLIGNMENT/GET_RAD_MEAS ==
  RadarParam : Inport
  RadarMeas : Inport  Port=2
  Bus Selector : BusSelector  OutputSignals=R1,R2,R3,R4,R5,R6
  Bus Selector1 : BusSelector  OutputSignals=RadarExtrinsics
  SnsrParam : Outport
  <R1> : Outport  Port=2
  <R2> : Outport  Port=3
  <R3> : Outport  Port=4
  <R4> : Outport  Port=5
  <R5> : Outport  Port=6
  <R6> : Outport  Port=7
  wires:
  Bus Selector/1 -> <R1>/1  "<R1>"
  Bus Selector/2 -> <R2>/1  "<R2>"
  Bus Selector/3 -> <R3>/1  "<R3>"
  Bus Selector/6 -> <R6>/1  "<R6>"
  Bus Selector/4 -> <R4>/1  "<R4>"
  Bus Selector/5 -> <R5>/1  "<R5>"
  RadarMeas/1 -> Bus Selector/1
  Bus Selector1/1 -> SnsrParam/1  "<RadarExtrinsics>"
  RadarParam/1 -> Bus Selector1/1

== system FusionMODEL_version4/OBJECT_TRACKER_SENSOR_FUSION/SPATIAL_ALLIGNMENT/RADAR_MEASUREMENTS_SPATIAL_ALLIGNMENT ==
  RadarCalibParam : Inport  BusOutputAsStruct=on
  R1 : Inport  Port=2
  R2 : Inport  Port=3
  R3 : Inport  Port=4
  R4 : Inport  Port=5
  R5 : Inport  Port=6
  R6 : Inport  Port=7
  RADAR_MEASUREMENTS_SPATIAL_ALLIGNMENT : Subsystem  TreatAsAtomicUnit=on
  SET_MEASUREMENTS : Subsystem
  StartingIndexes1 : Subsystem
  RadarMeasTransformed : Outport
  wires:
  StartingIndexes1/1(StartingIndexes) -> RADAR_MEASUREMENTS_SPATIAL_ALLIGNMENT/2(RadarStartingIdx)
  R1/1 -> RADAR_MEASUREMENTS_SPATIAL_ALLIGNMENT/3(R1)
  R2/1 -> RADAR_MEASUREMENTS_SPATIAL_ALLIGNMENT/4(R2)
  R4/1 -> RADAR_MEASUREMENTS_SPATIAL_ALLIGNMENT/6(R4)
  R5/1 -> RADAR_MEASUREMENTS_SPATIAL_ALLIGNMENT/7(R5)
  RadarCalibParam/1 -> RADAR_MEASUREMENTS_SPATIAL_ALLIGNMENT/1(RadarCallibrationParam), StartingIndexes1/1(SnsrCallib)
  R6/1 -> RADAR_MEASUREMENTS_SPATIAL_ALLIGNMENT/8(R6)
  R3/1 -> RADAR_MEASUREMENTS_SPATIAL_ALLIGNMENT/5(R3)
  RADAR_MEASUREMENTS_SPATIAL_ALLIGNMENT/1(RadarMeasTransformed) -> SET_MEASUREMENTS/1(CTSmeasMAT)
  RADAR_MEASUREMENTS_SPATIAL_ALLIGNMENT/4(MaxNoValidMeas) -> SET_MEASUREMENTS/4(validMeasCount)
  SET_MEASUREMENTS/1(CTSmeasMATout) -> RadarMeasTransformed/1
  RADAR_MEASUREMENTS_SPATIAL_ALLIGNMENT/2(RadarMeasCOVTransformed) -> SET_MEASUREMENTS/2(CTSCovMAT)
  RADAR_MEASUREMENTS_SPATIAL_ALLIGNMENT/3(RadarMeasRef) -> SET_MEASUREMENTS/3(CTSRefMAT)

== system FusionMODEL_version4/SENSOR_MEASUREMENTS/RADAR_CAMERA_EGO_SENSOR_INTERFACE/CameraSensors ==
  time : Inport
  nObjCamera : Inport  Port=2
  CAMSensorBUS : Inport  Port=3  OutDataTypeStr=Bus: CameraMeasParam  PortDimensions=200  BusOutputAsStruct=on
  Camera1 : Subsystem  TreatAsAtomicUnit=on
  Camera2 : Subsystem  TreatAsAtomicUnit=on
  Camera3 : Subsystem  TreatAsAtomicUnit=on
  Camera4 : Subsystem  TreatAsAtomicUnit=on
  Camera5 : Subsystem  TreatAsAtomicUnit=on
  Camera6 : Subsystem  TreatAsAtomicUnit=on
  Camera7 : Subsystem  TreatAsAtomicUnit=on
  Camera8 : Subsystem  TreatAsAtomicUnit=on
  C1 : Outport
  C2 : Outport  Port=2
  C3 : Outport  Port=3
  C4 : Outport  Port=4
  C5 : Outport  Port=5
  C6 : Outport  Port=6
  C7 : Outport  Port=7
  C8 : Outport  Port=8
  wires:
  CAMSensorBUS/1 -> Camera1/3(SensorMeas), Camera2/3(SensorMeas), Camera3/3(SensorMeas), Camera4/3(SensorMeas), Camera6/3(SensorMeas), Camera8/3(SensorMeas), Camera7/3(SensorMeas), Camera5/3(SensorMeas)
  nObjCamera/1 -> Camera4/2(nObjCamera), Camera6/2(nObjCamera), Camera8/2(nObjCamera), Camera7/2(nObjCamera), Camera5/2(nObjCamera), Camera3/2(nObjCamera), Camera2/2(nObjCamera), Camera1/2(nObjCamera)
  Camera1/1(C1) -> C1/1
  time/1 -> Camera1/1(timeIdx), Camera4/1(timeIdx), Camera5/1(timeIdx), Camera6/1(timeIdx), Camera8/1(timeIdx), Camera7/1(timeIdx), Camera3/1(timeIdx), Camera2/1(timeIdx)
  Camera4/1(C4) -> C4/1
  Camera3/1(C3) -> C3/1
  Camera6/1(C6) -> C6/1
  Camera5/1(C5) -> C5/1
  Camera2/1(C2) -> C2/1
  Camera7/1(C7) -> C7/1
  Camera8/1(C8) -> C8/1

== system FusionMODEL_version4/SENSOR_MEASUREMENTS/RADAR_CAMERA_EGO_SENSOR_INTERFACE/Clock ==
  note: A n Array Of maximum number of sensor measurements for each Radar
  note: A n Array Of maximum number of sensor measurements for each Camera
  Add : Sum
  Constant : Constant
  Constant1 : Constant  Value=RAD_nMeas
  Constant2 : Constant  Value=CAM_nMeas
  Constant3 : Constant  Value=int32([2, 2, 2, 2, 2, 2, 2, 2])
  Data Type Conversion : DataTypeConversion  OutDataTypeStr=int16
  Digital Clock : DigitalClock  SampleTime=SamplingTime
  Gain : Gain  Gain=1/SamplingTime
  time : Outport
  nObjRadar : Outport  Port=2
  nObjCamera : Outport  Port=3
  nLinesCamera : Outport  Port=4
  wires:
  Digital Clock/1 -> Gain/1
  Gain/1 -> Add/1
  Add/1 -> Data Type Conversion/1
  Constant/1 -> Add/2
  Data Type Conversion/1 -> time/1
  Constant1/1 -> nObjRadar/1
  Constant2/1 -> nObjCamera/1
  Constant3/1 -> nLinesCamera/1

== system FusionMODEL_version4/SENSOR_MEASUREMENTS/RADAR_CAMERA_EGO_SENSOR_INTERFACE/EgoSensors ==
  timeIdx : Inport
  In1 : Inport  Port=2  OutDataTypeStr=Bus: EGO_PARAM  PortDimensions=1
  Assignment : Assignment  DiagnosticForDimensions=Warning  IndexOptions=Index vector (dialog)  Indices=1  OutputSizes=1
  Bus Creator : BusCreator  Inputs=7  OutDataTypeStr=Bus: EGO_PARAM  NonVirtualBus=on
  ExtractMeasParam : Subsystem
  EgoSensorData : Outport
  EgoIgnitionStatus : Outport  Port=2
  wires:
  timeIdx/1 -> ExtractMeasParam/1(timeIdx)
  Bus Creator/1 -> Assignment/2
  Assignment/1 -> EgoSensorData/1
  ExtractMeasParam/1(EgoTimeStamp) -> Bus Creator/1  "TimeStamp"
  ExtractMeasParam/2(EgoPx) -> Bus Creator/2  "px"
  ExtractMeasParam/3(EgoPy) -> Bus Creator/3  "py"
  ExtractMeasParam/4(EgoVx) -> Bus Creator/4  "vx"
  ExtractMeasParam/6(EgoYaw) -> Bus Creator/6  "yaw"
  ExtractMeasParam/7(EgoYawRate) -> Bus Creator/7  "yawRate"
  ExtractMeasParam/5(EgoVy) -> Bus Creator/5  "vy"
  In1/1 -> Assignment/1
  ExtractMeasParam/8(EgoIgnitionStatus) -> EgoIgnitionStatus/1

== system FusionMODEL_version4/SENSOR_MEASUREMENTS/RADAR_CAMERA_EGO_SENSOR_INTERFACE/RadarSensors ==
  time : Inport
  nObjRadar : Inport  Port=2
  RADSensorBUS : Inport  Port=3  OutDataTypeStr=Bus: RadarMeasParam  PortDimensions=200  BusOutputAsStruct=on
  Radar1 : Subsystem  TreatAsAtomicUnit=on
  Radar2 : Subsystem  TreatAsAtomicUnit=on
  Radar3 : Subsystem  TreatAsAtomicUnit=on
  Radar4 : Subsystem  TreatAsAtomicUnit=on
  Radar5 : Subsystem  TreatAsAtomicUnit=on
  Radar6 : Subsystem  TreatAsAtomicUnit=on
  R1 : Outport
  R2 : Outport  Port=2
  R3 : Outport  Port=3
  R4 : Outport  Port=4
  R5 : Outport  Port=5
  R6 : Outport  Port=6
  wires:
  RADSensorBUS/1 -> Radar2/3(SensorMeas), Radar6/3(SensorMeas), Radar5/3(SensorMeas), Radar4/3(SensorMeas), Radar3/3(SensorMeas), Radar1/3(SensorMeas)
  nObjRadar/1 -> Radar3/2(nObjRadar), Radar6/2(nObjRadar), Radar5/2(nObjRadar), Radar4/2(nObjRadar), Radar2/2(nObjRadar), Radar1/2(nObjRadar)
  Radar1/1(R1) -> R1/1
  time/1 -> Radar3/1(timeIdx), Radar6/1(timeIdx), Radar5/1(timeIdx), Radar4/1(timeIdx), Radar2/1(timeIdx), Radar1/1(timeIdx)
  Radar4/1(R4) -> R4/1
  Radar3/1(R3) -> R3/1
  Radar6/1(R6) -> R6/1
  Radar5/1(R5) -> R5/1
  Radar2/1(R2) -> R2/1

== system FusionMODEL_version4/SENSOR_MEASUREMENTS/RADAR_CAMERA_EGO_SENSOR_INTERFACE/RoadSensors ==
  time : Inport
  nLinesCamera : Inport  Port=2
  CameraLineCoeff1 : Inport  Port=3  OutDataTypeStr=Bus: LineMeasParam  PortDimensions=10
  Camera1 : Subsystem  TreatAsAtomicUnit=on
  Camera2 : Subsystem  TreatAsAtomicUnit=on
  Camera3 : Subsystem  TreatAsAtomicUnit=on
  Camera4 : Subsystem  TreatAsAtomicUnit=on
  Camera5 : Subsystem  TreatAsAtomicUnit=on
  Camera6 : Subsystem  TreatAsAtomicUnit=on
  Camera7 : Subsystem  TreatAsAtomicUnit=on
  Camera8 : Subsystem  TreatAsAtomicUnit=on
  C1 : Outport
  C2 : Outport  Port=2
  C3 : Outport  Port=3
  C4 : Outport  Port=4
  C5 : Outport  Port=5
  C6 : Outport  Port=6
  C7 : Outport  Port=7
  C8 : Outport  Port=8
  wires:
  Camera2/1(C1) -> C2/1
  Camera7/1(C1) -> C7/1
  CameraLineCoeff1/1 -> Camera1/3(CameraLineCoeff), Camera2/3(CameraLineCoeff), Camera3/3(CameraLineCoeff), Camera4/3(CameraLineCoeff), Camera5/3(CameraLineCoeff), Camera6/3(CameraLineCoeff), Camera8/3(CameraLineCoeff), Camera7/3(CameraLineCoeff)
  time/1 -> Camera1/1(timeIdx), Camera2/1(timeIdx), Camera3/1(timeIdx), Camera4/1(timeIdx), Camera5/1(timeIdx), Camera6/1(timeIdx), Camera8/1(timeIdx), Camera7/1(timeIdx)
  Camera1/1(C1) -> C1/1
  Camera6/1(C1) -> C6/1
  Camera5/1(C1) -> C5/1
  Camera8/1(C1) -> C8/1
  nLinesCamera/1 -> Camera2/2(nLines), Camera3/2(nLines), Camera4/2(nLines), Camera5/2(nLines), Camera6/2(nLines), Camera8/2(nLines), Camera7/2(nLines), Camera1/2(nLines)
  Camera3/1(C1) -> C3/1
  Camera4/1(C1) -> C4/1

== system FusionMODEL_version4/OBJECT_TRACKER_SENSOR_FUSION/NEAREST_NEIGHBOUR_FOR_CAMERA_MEASUREMENT_GROUPING/NN_MEASUREMENT_GROUPING_WITHIN_EPS/COMPUTE_MEAN_IF_CLUSTER_FORMED ==
  meas : Inport
  CLSTR_DATA : Inport  Port=2
  Enable : EnablePort
  COMPUTE_COVARIANCE1 : Subsystem
  COMPUTE_COVARIANCE_SUM : Subsystem  TreatAsAtomicUnit=on
  COMPUTE_MEAN : Subsystem
  COMPUTE_MEAN_SUM : Subsystem  TreatAsAtomicUnit=on
  GET_DATA : Subsystem
  CLSTR_CNTR_UPD : Outport
  CLSTR_COV_UPD : Outport  Port=2
  wires:
  GET_DATA/1(nPts) -> [nPts], COMPUTE_MEAN_SUM/2(nPoints), COMPUTE_MEAN/2(n), COMPUTE_COVARIANCE_SUM/3(nPoints)
  GET_DATA/2(<ClusterMember>) -> COMPUTE_COVARIANCE_SUM/4(ClusterMembers), [ClstrMembers]
  [Meas] -> COMPUTE_COVARIANCE_SUM/2(MeasArray)
  meas/1 -> [Meas], COMPUTE_MEAN_SUM/3(MeasArray)
  [ClstrMembers] -> COMPUTE_MEAN_SUM/1(ClusterMembers)
  COMPUTE_COVARIANCE1/1(Covariance) -> CLSTR_COV_UPD/1
  [nPts] -> COMPUTE_COVARIANCE1/2(n)
  COMPUTE_MEAN/1(mean) -> CLSTR_CNTR_UPD/1, COMPUTE_COVARIANCE_SUM/1(mean)
  CLSTR_DATA/1 -> GET_DATA/1(CLSTR)
  COMPUTE_MEAN_SUM/1(ClusterMeanSUM) -> COMPUTE_MEAN/1(mean_sum)
  COMPUTE_COVARIANCE_SUM/1(ClusterCovSUM) -> COMPUTE_COVARIANCE1/1(covariance_sum)

== system FusionMODEL_version4/OBJECT_TRACKER_SENSOR_FUSION/NEAREST_NEIGHBOUR_FOR_CAMERA_MEASUREMENT_GROUPING/NN_MEASUREMENT_GROUPING_WITHIN_EPS/For Iterator Subsystem ==
  idx_i : Inport
  measArray : Inport  Port=2
  CLSTR_DATA : Inport  Port=3
  If : If  IfExpression=u1 ~= 0
  If Action Subsystem : Subsystem  TreatAsAtomicUnit=on
  MERGE_SIGNALS : Subsystem
  NN : Subsystem
  Subsystem : Subsystem
  nPts : Outport
  CLSTR_DATA_out : Outport  Port=2
  wires:
  idx_i/1 -> Subsystem/1(idx_i), NN/3(idx_i)
  CLSTR_DATA/1 -> Subsystem/2(CLSTR_in)
  Subsystem/1(isNotVisited) -> If/1
  If/1 -> NN/Action
  If/2 -> If Action Subsystem/Action
  measArray/1 -> NN/2(measArray)
  If Action Subsystem/1(CLSTR_DATA_NO_UPD) -> MERGE_SIGNALS/1(CLSTR_NO_UPD)
  If Action Subsystem/2(nPtsEpsNoUpd) -> MERGE_SIGNALS/2(nPtsEpsNoUpd)
  NN/1(nPtsEps) -> MERGE_SIGNALS/3(nPtsUpd)
  MERGE_SIGNALS/2(CLSTR_DATA) -> CLSTR_DATA_out/1
  Subsystem/2(CLSTR_out) -> NN/1(CLSTR_DATA), If Action Subsystem/1(CLSTR_DATA)
  NN/2(CLSTR_DATA_UPD) -> MERGE_SIGNALS/4(CLSTR_UPD)
  MERGE_SIGNALS/1(nPtsEps) -> nPts/1

== system FusionMODEL_version4/OBJECT_TRACKER_SENSOR_FUSION/NEAREST_NEIGHBOUR_FOR_CAMERA_MEASUREMENT_GROUPING/NN_MEASUREMENT_GROUPING_WITHIN_EPS/Subsystem1 ==
  CLSTR_DATA : Inport
  Constant : Constant  Value=uint16(0)
  GreaterThan : RelationalOperator  Operator=>  OutDataTypeStr=boolean  RndMeth=Simplest
  Logical Operator : Logic  Operator=NOT  AllPortsSameDT=off  OutDataTypeStr=boolean
  NoUpd : Outport
  Upd : Outport  Port=2
  wires:
  CLSTR_DATA/1 -> GreaterThan/1
  GreaterThan/1 -> Logical Operator/1, Upd/1
  Constant/1 -> GreaterThan/2
  Logical Operator/1 -> NoUpd/1

== system FusionMODEL_version4/OBJECT_TRACKER_SENSOR_FUSION/NEAREST_NEIGHBOUR_FOR_CAMERA_MEASUREMENT_GROUPING/NN_MEASUREMENT_GROUPING_WITHIN_EPS/Subsystem2 ==
  Enable : EnablePort
  Constant : Constant  Value=single(zeros(2,1))  VectorParams1D=off
  Constant1 : Constant  Value=single(zeros(2,2))  VectorParams1D=off
  Mean : Outport
  Cov : Outport  Port=2
  wires:
  Constant/1 -> Mean/1
  Constant1/1 -> Cov/1

== system FusionMODEL_version4/OBJECT_TRACKER_SENSOR_FUSION/NEAREST_NEIGHBOUR_FOR_CAMERA_MEASUREMENT_GROUPING/NN_MEASUREMENT_GROUPING_WITHIN_EPS/Subsystem3 ==
  MeanNoUpd : Inport
  CovNoUpd : Inport  Port=2
  MeanUpd : Inport  Port=3
  CovUpd : Inport  Port=4
  CLSTR_DATA : Inport  Port=5
  Flag : Inport  Port=6
  GET_DATA_FROM_BUS : Subsystem
  SET_DATA_TO_BUS : Subsystem
  UPDATE_CLUSTER_DATA : Subsystem
  CLSTR_DATA_UPD : Outport
  wires:
  GET_DATA_FROM_BUS/1(<ClusterCenter>) -> UPDATE_CLUSTER_DATA/1(Center_ARRAY)
  GET_DATA_FROM_BUS/2(<ClusterCovariance>) -> UPDATE_CLUSTER_DATA/2(Cov_ARRAY)
  GET_DATA_FROM_BUS/3(<nClusters>) -> UPDATE_CLUSTER_DATA/3(ID)
  UPDATE_CLUSTER_DATA/1(CenterUpd) -> SET_DATA_TO_BUS/2(Mean_ARRAY)
  UPDATE_CLUSTER_DATA/2(CovUpd) -> SET_DATA_TO_BUS/3(Cov_ARRAY)
  MeanUpd/1 -> UPDATE_CLUSTER_DATA/4(mean1)
  MeanNoUpd/1 -> UPDATE_CLUSTER_DATA/5(mean2)
  CovNoUpd/1 -> UPDATE_CLUSTER_DATA/7(Cov2)
  Flag/1 -> UPDATE_CLUSTER_DATA/8(FLAG)
  CovUpd/1 -> UPDATE_CLUSTER_DATA/6(Cov1)
  CLSTR_DATA/1 -> SET_DATA_TO_BUS/1(CLSTR_DATA), GET_DATA_FROM_BUS/1(CLSTR_DATA)
  SET_DATA_TO_BUS/1("CLSTR_DATA_UPD ") -> CLSTR_DATA_UPD/1

== system FusionMODEL_version4/OBJECT_TRACKER_SENSOR_FUSION/SENSOR_LAYOUT_AND_CHRACTERIZATION/PRE_COMPUTE_SENSOR_FOV_GRID/COMPUTE_CAMERA_SNSR_GRID ==
  GridIDVector : Inport
  GridParam : Inport  Port=2
  SnsrParam : Inport  Port=3
  ComputeCoverageANDConfidence : Subsystem  TreatAsAtomicUnit=on
  GET_SENSOR_PARAMETERS : Subsystem
  SENSOR_LOOP : ForIterator  ResetStates=reset  IterationLimit=nCameras  IterationVariableDataType=int8
  Unit Delay : UnitDelay  InitialCondition=RegionConfidenceCAM  SampleTime=-1
  Unit Delay1 : UnitDelay  InitialCondition=FOVOverlapCAM  SampleTime=-1
  Width : Width
  RegionConfidence : Outport
  FOVOverlap : Outport  Port=2
  wires:
  GridIDVector/1 -> ComputeCoverageANDConfidence/3(GridIDVector), Width/1
  Width/1 -> ComputeCoverageANDConfidence/2(nGridCells)
  SENSOR_LOOP/1 -> ComputeCoverageANDConfidence/5(SensorID), GET_SENSOR_PARAMETERS/1(SensorID)
  SnsrParam/1 -> GET_SENSOR_PARAMETERS/2(SensorParam)
  GET_SENSOR_PARAMETERS/1(extrinsic) -> ComputeCoverageANDConfidence/6(SensorExtrinsic)
  GET_SENSOR_PARAMETERS/2(intrinsic) -> ComputeCoverageANDConfidence/7(SensorIntrinsic)
  GridParam/1 -> ComputeCoverageANDConfidence/4(GridParam)
  ComputeCoverageANDConfidence/1(RegionConfidence) -> Unit Delay/1, RegionConfidence/1
  ComputeCoverageANDConfidence/2(FOVOverlap) -> Unit Delay1/1, FOVOverlap/1
  Unit Delay/1 -> ComputeCoverageANDConfidence/1(RegionConfidenceArray)
  Unit Delay1/1 -> ComputeCoverageANDConfidence/8(FOVOverlapArray)

== system FusionMODEL_version4/OBJECT_TRACKER_SENSOR_FUSION/SENSOR_LAYOUT_AND_CHRACTERIZATION/PRE_COMPUTE_SENSOR_FOV_GRID/COMPUTE_GRID_DIMENSION ==
  note: Set_Grid_Parameters
  note: Compute_number_of_grid_cells
  note: Compute_number_of_logitudinal_Grid_Cells
  note: Compute_number_of_lateral_Grid_Cells
  Bus Creator1 : BusCreator  Inputs=3
  Bus Creator2 : BusCreator  Inputs=4
  Bus Creator3 : BusCreator  Inputs=4
  Constant1 : Constant  Value=single(1)
  Constant3 : Constant  Value=single(1)
  Data Type Conversion : DataTypeConversion  OutDataTypeStr=int32
  Data Type Conversion1 : DataTypeConversion  OutDataTypeStr=uint32
  Data Type Conversion3 : DataTypeConversion  OutDataTypeStr=int32
  Divide : Product  Inputs=*/
  Divide1 : Product  Inputs=/*
  Divide2 : Product  Inputs=*/
  Divide3 : Product  Inputs=/*
  Floor{,1..3} (4 alike) : Rounding
  Gain : Gain  Gain=single(-1)
  Gain1 : Gain  Gain=single(-1)
  GridFrontLimit : Constant  Value=xFront
  GridLeftLimit : Constant  Value=yLeft
  GridRearLimit : Constant  Value=xRear
  GridResLat : Constant  Value=yRes
  GridResLong : Constant  Value=xRes
  GridRightLimit : Constant  Value=yRight
  Minus : Sum  Inputs=+-+
  Minus1 : Sum  Inputs=+-+
  Multiply : Product
  Saturation : Saturate  UpperLimit=10  LowerLimit=0.5
  Saturation1 : Saturate  UpperLimit=10  LowerLimit=0.5
  Cx : Outport
  Cy : Outport  Port=2
  GridParam : Outport  Port=3
  wires:
  GridResLong/1 -> Saturation/1
  Saturation/1 -> [xRes], Divide1/1, Divide/2
  GridFrontLimit/1 -> [xFront], Divide/1
  Divide/1 -> Floor/1
  GridRearLimit/1 -> Gain/1
  Gain/1 -> [xRear], Divide1/2
  Divide1/1 -> Floor1/1
  Floor/1 -> Minus/1
  Floor1/1 -> Minus/2
  Constant1/1 -> Minus/3
  Divide2/1 -> Floor2/1
  GridRightLimit/1 -> [yRight], Divide2/1
  GridResLat/1 -> Saturation1/1
  Constant3/1 -> Minus1/3
  Saturation1/1 -> [yRes], Divide3/1, Divide2/2
  GridLeftLimit/1 -> Gain1/1
  Gain1/1 -> [yLeft], Divide3/2
  Floor2/1 -> Minus1/1
  Divide3/1 -> Floor3/1
  Floor3/1 -> Minus1/2
  Minus/1 -> Multiply/1, Data Type Conversion/1
  Minus1/1 -> Multiply/2, Data Type Conversion3/1
  Data Type Conversion/1 -> [nGridCellsLong]
  Multiply/1 -> Data Type Conversion1/1
  Data Type Conversion1/1 -> [nGridCells]
  [nGridCells] -> Bus Creator1/1  "nGridCells"
  [nGridCellsLat] -> Cy/1, Bus Creator2/1  "nGridCellsLat"
  [yRes] -> Bus Creator2/2  "yRes"
  [yRight] -> Bus Creator2/3  "yRight"
  [yLeft] -> Bus Creator2/4  "yLeft"
  Bus Creator2/1 -> Bus Creator1/3  "yGridParameters"
  Data Type Conversion3/1 -> [nGridCellsLat]
  [nGridCellsLong] -> Cx/1, Bus Creator3/1  "nGridCellsLong"
  [xRear] -> Bus Creator3/4  "xRear"
  Bus Creator3/1 -> Bus Creator1/2  "xGridParameters"
  [xRes] -> Bus Creator3/2  "xRes"
  [xFront] -> Bus Creator3/3  "xFront"
  Bus Creator1/1 -> GridParam/1

== system FusionMODEL_version4/OBJECT_TRACKER_SENSOR_FUSION/SENSOR_LAYOUT_AND_CHRACTERIZATION/PRE_COMPUTE_SENSOR_FOV_GRID/COMPUTE_RADAR_SNSR_GRID ==
  SnsrParam : Inport
  GridParam : Inport  Port=2
  GridIDVector : Inport  Port=3
  ComputeCoverageANDConfidence : Subsystem  TreatAsAtomicUnit=on
  GET_SENSOR_PARAMETERS : Subsystem
  SENSOR_LOOP : ForIterator  ResetStates=reset  IterationLimit=nRadars  IterationVariableDataType=int8
  Unit Delay : UnitDelay  InitialCondition=RegionConfidenceRAD  SampleTime=-1
  Unit Delay1 : UnitDelay  InitialCondition=FOVOverlapRAD  SampleTime=-1
  Width : Width
  RegionConfidence : Outport
  FOVOverlap : Outport  Port=2
  wires:
  GridIDVector/1 -> ComputeCoverageANDConfidence/3(GridIDVector), Width/1
  Width/1 -> ComputeCoverageANDConfidence/2(nGridCells)
  SENSOR_LOOP/1 -> ComputeCoverageANDConfidence/5(SensorID), GET_SENSOR_PARAMETERS/1(SensorID)
  SnsrParam/1 -> GET_SENSOR_PARAMETERS/2(SensorParam)
  GET_SENSOR_PARAMETERS/1(extrinsic) -> ComputeCoverageANDConfidence/6(SensorExtrinsic)
  GET_SENSOR_PARAMETERS/2(intrinsic) -> ComputeCoverageANDConfidence/7(SensorIntrinsic)
  GridParam/1 -> ComputeCoverageANDConfidence/4(GridParam)
  ComputeCoverageANDConfidence/1(RegionConfidence) -> Unit Delay/1, RegionConfidence/1
  ComputeCoverageANDConfidence/2(FOVOverlap) -> Unit Delay1/1, FOVOverlap/1
  Unit Delay/1 -> ComputeCoverageANDConfidence/1(RegionConfidenceArray)
  Unit Delay1/1 -> ComputeCoverageANDConfidence/8(FOVOverlapArray)
